simulink model "MutantsModel2"  (R2017b)
settings: Solver=ode3  StartTime=0.0  StopTime=inf  FixedStep=ts  RelTol=0.01  EnableMultiTasking=on
InitFcn:
  | ts=0.0005
  | %ts=100e-6;
StartFcn:
  | close all
StopFcn:
  | % Speed Torque Characterstic
  | 
  | 
  | %figure('Units','pixels', ...
  | %'Color',[1 1 1], ...
  | %'Name','Speed Torque Characterstic',...
  | %'NumberTitle','off',...
  | %'Position',[400 50 470 300], ...
  | %'ToolBar','none');
  | 
  | 
  | 
  | %plot(N_pi,Te_pi)
  | %title('Speed Torque Characterstic')
  | %xlabel('Speed [ RPM ]')
  | %ylabel('Electromagnetic Te_pi [ Nm ] ')
  | %grid on
  | %clear p4 p7 param5 param6 param8 parametres visible voltage
  | 
  | 
  | %clc
values from neighbouring files (symbols this model uses):
  TestOrder = [i]    [ExecuteTestSuite.m]    (also in mutants.m)
undefined symbols (not defined in the file or in its folder): emergency_button2, emergency_buttons, tc_simul, tc_size, temperature, trans1, trans2, trans3, trans4
libraries: simulink x44, powerlib_extras x11
(part 2 of 5)

== system MutantsModel2/mutant1/PI Control1 ==
  N* : Inport
  N : Inport  Port=2
  Abs : Abs  SaturateOnIntegerOverflow=on
  Abs1 : Abs  SaturateOnIntegerOverflow=on
  Abs2 : Abs
  Compare To Constant : simulink/Logic and Bit Operations/Compare To Constant  relop=<=  const=0.1  OutDataTypeStr=uint8
  Constant : Constant  Value=0
  Divide : Product  Inputs=/*
  Integrator Limited : Integrator  LimitOutput=on  UpperSaturationLimit=30  LowerSaturationLimit=-30
  Proportional gain : Gain  Gain=0.8  SaturateOnIntegerOverflow=on  OutDataTypeStr=Inherit: Same as input  ParamDataTypeStr=Inherit: Same as input
  Rate Transition3 : RateTransition  OutPortSampleTimeOpt=Inherit
  Saturation : Saturate  UpperLimit=inf  LowerLimit=2
  Saturation2 : Saturate  UpperLimit=120  LowerLimit=0.02
  Sum1 : Sum  Inputs=|+-  SaturateOnIntegerOverflow=on  InputSameDT=on  OutDataTypeStr=Inherit: Same as first input
  Sum2 : Sum  SaturateOnIntegerOverflow=on  InputSameDT=on  OutDataTypeStr=Inherit: Same as first input
  Sum3 : Sum  Inputs=|++  SaturateOnIntegerOverflow=on  InputSameDT=on  OutDataTypeStr=Inherit: Same as first input
  Switch : Switch  Threshold=0.5
  ctrl_sat : Saturate  UpperLimit=30  LowerLimit=-30
  rpm2hz : Gain  Gain=4/120  SaturateOnIntegerOverflow=on  OutDataTypeStr=Inherit: Same as input  ParamDataTypeStr=Inherit: Same as input
  "rpm2hz  " : Gain  Gain=4/120  SaturateOnIntegerOverflow=on  OutDataTypeStr=Inherit: Same as input  ParamDataTypeStr=Inherit: Same as input
  Freq* : Outport
  wires:
  N*/1 -> rpm2hz/1
  Sum2/1 -> ctrl_sat/1
  Sum3/1 -> Saturation2/1
  ctrl_sat/1 -> Sum3/1
  rpm2hz/1 -> Abs/1
  Proportional gain/1 -> Sum2/2
  "rpm2hz  "/1 -> Abs1/1
  Saturation2/1 -> Rate Transition3/1
  Sum1/1 -> Proportional gain/1, Switch/1, Abs2/1
  Abs/1 -> Saturation/1, Sum1/1
  Rate Transition3/1 -> Freq*/1
  Abs1/1 -> Sum3/2, Sum1/2
  N/1 -> "rpm2hz  "/1
  Integrator Limited/1 -> Sum2/1
  Divide/1 -> Compare To Constant/1
  Abs2/1 -> Divide/2
  Compare To Constant/1 -> Switch/2
  Constant/1 -> Switch/3
  Switch/1 -> Integrator Limited/1
  Saturation/1 -> Divide/1

== system MutantsModel2/mutant1/Subsystem ==
  Speed : Inport
  EmergButton1 : Inport  Port=2
  EmergButton2 : Inport  Port=3
  Temperature : Inport  Port=4
  Compare To Constant : simulink/Logic and Bit Operations/Compare To Constant  relop=>  const=100  OutDataTypeStr=boolean
  Compare To Constant1 : simulink/Logic and Bit Operations/Compare To Constant  relop===  const=0  OutDataTypeStr=boolean
  Constant : Constant  Value=emergency_buttons
  Constant1 : Constant  Value=temperature
  Constant2 : Constant  Value=emergency_button2
  Ir_a3 : Scope
  Logical Operator : Logic  Operator=OR  AllPortsSameDT=off  OutDataTypeStr=boolean
  Logical Operator1 : Logic  AllPortsSameDT=off  OutDataTypeStr=boolean
  Logical Operator2 : Logic  AllPortsSameDT=off  OutDataTypeStr=boolean
  Logical Operator3 : Logic  AllPortsSameDT=off  OutDataTypeStr=boolean
  Speed_to_0 : Constant  Value=0
  Switch : Switch  Criteria=u2 ~= 0
  Switch1 : Switch  Criteria=u2 ~= 0
  Switch2 : Switch  Criteria=u2 ~= 0
  Transfer Fcn1 : TransferFcn  Denominator=[10 1]
  "MotorSpeed " : Outport
  wires:
  Transfer Fcn1/1 -> Switch/3
  Compare To Constant1/1 -> Switch2/2
  Switch2/1 -> "MotorSpeed "/1, Ir_a3/1
  Switch1/1 -> Compare To Constant1/1, Switch2/1, Switch2/3
  Constant2/1 -> Logical Operator3/2
  Logical Operator3/1 -> Logical Operator/2
  Logical Operator2/1 -> Switch1/2
  Constant1/1 -> Logical Operator2/2
  Compare To Constant/1 -> Logical Operator2/1
  Temperature/1 -> Compare To Constant/1
  Constant/1 -> Logical Operator1/2
  Logical Operator1/1 -> Switch/2
  Speed_to_0/1 -> Switch/1, Switch1/1
  Switch/1 -> Switch1/3
  Speed/1 -> Transfer Fcn1/1
  Logical Operator/1 -> Logical Operator1/1
  EmergButton2/1 -> Logical Operator3/1
  EmergButton1/1 -> Logical Operator/1

== system MutantsModel2/mutant1/VSI ==
  Freq : Inport
  Fcn : Fcn  Expr=(2*sqrt(2/3)*Vdc/3)*(2*u(1)-u(2)-u(3))
  Fcn1 : Fcn  Expr=(2*sqrt(2/3)*Vdc/3)*(2*u(2)-u(3)-u(1))
  Fcn2 : Fcn  Expr=(2*sqrt(2/3)*Vdc/3)*(2*u(3)-u(2)-u(1))
  SPWM : Subsystem
  Va : Outport
  Vb : Outport  Port=2
  Vc : Outport  Port=3
  wires:
  Freq/1 -> SPWM/1(Freq)
  Fcn/1 -> Va/1
  Fcn2/1 -> Vc/1
  Fcn1/1 -> Vb/1
  SPWM/1(g) -> Fcn1/1, Fcn/1, Fcn2/1

== system MutantsModel2/mutant10/1 HP , 220 V Induction Motor ==
  tau : Inport
  V_a : Inport  Port=2
  V_b : Inport  Port=3
  V_c : Inport  Port=4
  Flux : Subsystem
  Measurements : Subsystem
  Mechanical : Subsystem
  Mux : Mux  Inputs=3
  Mux1 : Mux  Inputs=3
  abc to dq : Subsystem
  d_block : Subsystem
  dq to abc : Subsystem
  "dq to abc " : Subsystem
  q_block : Subsystem
  rad2rpm : Gain  Gain=30/pi
  m : Outport
  wires:
  Measurements/1(m) -> m/1
  rad2rpm/1 -> Measurements/8(N)
  Mux1/1 -> Measurements/2(I_r)
  Mux/1 -> Measurements/1(I_s)
  "dq to abc "/2(i_rb) -> Mux1/2
  "dq to abc "/3(i_rc) -> Mux1/3
  dq to abc/3(i_sc) -> Mux/3
  dq to abc/2(i_sb) -> Mux/2
  "dq to abc "/1(i_ra) -> Mux1/1
  dq to abc/1(i_sa) -> Mux/1
  V_a/1 -> abc to dq/1(Va)
  V_b/1 -> abc to dq/2(Vb)
  V_c/1 -> abc to dq/3(Vc)
  abc to dq/2(V_qs) -> Flux/2(V_qs)
  abc to dq/1(V_ds) -> Flux/1(V_ds)
  Flux/3(shi_qs) -> Mechanical/2(shi_qs), q_block/1(shi_qs)
  Flux/2("shi_dr ") -> d_block/2(shi_dr)
  tau/1 -> Mechanical/5(tau)
  Mechanical/1(Te) -> Measurements/7(Te)
  q_block/1(i_qs) -> Flux/5(I_qs), dq to abc/2(I_q), Measurements/5(I_qs), Measurements/4(I_dr), Mechanical/4(i_qs)
  q_block/2(i_qr) -> Flux/6(I_qr), "dq to abc "/2(I_q), Measurements/6(I_qr)
  d_block/2(i_dr) -> "dq to abc "/1(I_d), Flux/4(I_dr)
  d_block/1(i_ds) -> Flux/3(I_ds), dq to abc/1(I_d), Measurements/3(I_ds), Mechanical/3(i_ds)
  Flux/4("shi_qr ") -> q_block/2(shi_qr)
  Flux/1(shi_ds) -> Mechanical/1(shi_ds), d_block/1(shi_ds)
  Mechanical/3(we) -> Flux/7(we)
  Mechanical/2(omegaR) -> rad2rpm/1

== system MutantsModel2/mutant10/Data Acquision ==
  note: DONE TO HAVE AN ALLOWABLE SIMULATION TIME
  m : Inport
  speed : Inport  Port=2
  2nd-Order Filter : powerlib_extras/Control  Blocks/2nd-Order Filter  FilterType=Lowpass  Fo=120  Zeta=0.707  Initialize=off  Vac_Init=[1 45 60]  Vdc_Init=-0.5  PlotResponse=off  param1=[1 500 1]
  Bus Selector : BusSelector  OutputSignals=Mechanical.Rotor Speed in (rpm),Mechanical.Electromagnetic Torque (N*m),Stator Measurement.Stator Current i_sa (A)
  Mux : Mux  Inputs=2
  filtroPasaBajos : TransferFcn  Denominator=[1 1]
  is_a : Outport
  Te(Nm) : Outport  Port=2
  wm : Outport  Port=3
  wm1 : Outport  Port=4
  wires:
  filtroPasaBajos/1 -> Mux/1, wm1/1
  Mux/1 -> wm/1
  speed/1 -> Mux/2
  Bus Selector/3 -> is_a/1  "<Stator Current i_sa (A)>"
  Bus Selector/1 -> filtroPasaBajos/1  "<Rotor Speed in (rpm)>"
  m/1 -> Bus Selector/1
  Bus Selector/2 -> 2nd-Order Filter/1  "<Electromagnetic Torque (N*m)>"
  2nd-Order Filter/1 -> Te(Nm)/1

== system MutantsModel2/mutant10/PI Control1 ==
  N* : Inport
  N : Inport  Port=2
  Abs : Abs  SaturateOnIntegerOverflow=on
  Abs1 : Abs  SaturateOnIntegerOverflow=on
  Abs2 : Abs
  Compare To Constant : simulink/Logic and Bit Operations/Compare To Constant  relop=<=  const=0.1  OutDataTypeStr=uint8
  Constant : Constant  Value=0
  Divide : Product  Inputs=/*
  Integrator Limited : Integrator  LimitOutput=on  UpperSaturationLimit=30  LowerSaturationLimit=-30
  Proportional gain : Gain  Gain=0.8  SaturateOnIntegerOverflow=on  OutDataTypeStr=Inherit: Same as input  ParamDataTypeStr=Inherit: Same as input
  Rate Transition3 : RateTransition  OutPortSampleTimeOpt=Inherit
  Saturation : Saturate  UpperLimit=inf  LowerLimit=2
  Saturation2 : Saturate  UpperLimit=120  LowerLimit=0.02
  Sum1 : Sum  Inputs=|+-  SaturateOnIntegerOverflow=on  InputSameDT=on  OutDataTypeStr=Inherit: Same as first input
  Sum2 : Sum  SaturateOnIntegerOverflow=on  InputSameDT=on  OutDataTypeStr=Inherit: Same as first input
  Sum3 : Sum  Inputs=|++  SaturateOnIntegerOverflow=on  InputSameDT=on  OutDataTypeStr=Inherit: Same as first input
  Switch : Switch  Threshold=0.5
  ctrl_sat : Saturate  UpperLimit=30  LowerLimit=-30
  rpm2hz : Gain  Gain=4/120  SaturateOnIntegerOverflow=on  OutDataTypeStr=Inherit: Same as input  ParamDataTypeStr=Inherit: Same as input
  "rpm2hz  " : Gain  Gain=4/120  SaturateOnIntegerOverflow=on  OutDataTypeStr=Inherit: Same as input  ParamDataTypeStr=Inherit: Same as input
  Freq* : Outport
  wires:
  N*/1 -> rpm2hz/1
  Sum2/1 -> ctrl_sat/1
  Sum3/1 -> Saturation2/1
  ctrl_sat/1 -> Sum3/1
  rpm2hz/1 -> Abs/1
  Proportional gain/1 -> Sum2/2
  "rpm2hz  "/1 -> Abs1/1
  Saturation2/1 -> Rate Transition3/1
  Sum1/1 -> Proportional gain/1, Switch/1, Abs2/1
  Abs/1 -> Saturation/1, Sum1/1
  Rate Transition3/1 -> Freq*/1
  Abs1/1 -> Sum3/2, Sum1/2
  N/1 -> "rpm2hz  "/1
  Integrator Limited/1 -> Sum2/1
  Divide/1 -> Compare To Constant/1
  Abs2/1 -> Divide/2
  Compare To Constant/1 -> Switch/2
  Constant/1 -> Switch/3
  Switch/1 -> Integrator Limited/1
  Saturation/1 -> Divide/1

== system MutantsModel2/mutant10/Subsystem ==
  Speed : Inport
  EmergButton1 : Inport  Port=2
  EmergButton2 : Inport  Port=3
  Temperature : Inport  Port=4
  Compare To Constant : simulink/Logic and Bit Operations/Compare To Constant  relop=>  const=100  OutDataTypeStr=boolean
  Compare To Constant1 : simulink/Logic and Bit Operations/Compare To Constant  relop===  const=0  OutDataTypeStr=boolean
  Constant : Constant  Value=emergency_buttons
  Constant1 : Constant  Value=temperature
  Constant2 : Constant  Value=emergency_button2
  Ir_a3 : Scope
  Logical Operator : Logic  Operator=OR  AllPortsSameDT=off  OutDataTypeStr=boolean
  Logical Operator1 : Logic  Operator=NAND  AllPortsSameDT=off  OutDataTypeStr=boolean
  Logical Operator2 : Logic  AllPortsSameDT=off  OutDataTypeStr=boolean
  Logical Operator3 : Logic  AllPortsSameDT=off  OutDataTypeStr=boolean
  Speed_to_0 : Constant  Value=0
  Switch : Switch  Criteria=u2 ~= 0
  Switch1 : Switch  Criteria=u2 ~= 0
  Switch2 : Switch  Criteria=u2 ~= 0
  Transfer Fcn1 : TransferFcn  Denominator=[20 1]
  "MotorSpeed " : Outport
  wires:
  Transfer Fcn1/1 -> Switch/3
  Compare To Constant1/1 -> Switch2/2
  Switch2/1 -> "MotorSpeed "/1, Ir_a3/1
  Switch1/1 -> Compare To Constant1/1, Switch2/1, Switch2/3
  Constant2/1 -> Logical Operator3/2
  Logical Operator3/1 -> Logical Operator/2
  Logical Operator2/1 -> Switch1/2
  Constant1/1 -> Logical Operator2/2
  Compare To Constant/1 -> Logical Operator2/1
  Temperature/1 -> Compare To Constant/1
  Constant/1 -> Logical Operator1/2
  Logical Operator1/1 -> Switch/2
  Speed_to_0/1 -> Switch/1, Switch1/1
  Switch/1 -> Switch1/3
  Speed/1 -> Transfer Fcn1/1
  Logical Operator/1 -> Logical Operator1/1
  EmergButton2/1 -> Logical Operator3/1
  EmergButton1/1 -> Logical Operator/1

== system MutantsModel2/mutant10/VSI ==
  Freq : Inport
  Fcn : Fcn  Expr=(2*sqrt(2/3)*Vdc/3)*(2*u(1)-u(2)-u(3))
  Fcn1 : Fcn  Expr=(2*sqrt(2/3)*Vdc/3)*(2*u(2)-u(3)-u(1))
  Fcn2 : Fcn  Expr=(2*sqrt(2/3)*Vdc/3)*(2*u(3)-u(2)-u(1))
  SPWM : Subsystem
  Va : Outport
  Vb : Outport  Port=2
  Vc : Outport  Port=3
  wires:
  Freq/1 -> SPWM/1(Freq)
  Fcn/1 -> Va/1
  Fcn2/1 -> Vc/1
  Fcn1/1 -> Vb/1
  SPWM/1(g) -> Fcn1/1, Fcn/1, Fcn2/1

== system MutantsModel2/mutant2/1 HP , 220 V Induction Motor ==
  tau : Inport
  V_a : Inport  Port=2
  V_b : Inport  Port=3
  V_c : Inport  Port=4
  Flux : Subsystem
  Measurements : Subsystem
  Mechanical : Subsystem
  Mux : Mux  Inputs=3
  Mux1 : Mux  Inputs=3
  abc to dq : Subsystem
  d_block : Subsystem
  dq to abc : Subsystem
  "dq to abc " : Subsystem
  q_block : Subsystem
  rad2rpm : Gain  Gain=30/pi
  m : Outport
  wires:
  Mechanical/2(omegaR) -> rad2rpm/1
  Mechanical/3(we) -> Flux/7(we)
  Flux/1(shi_ds) -> d_block/1(shi_ds), Mechanical/1(shi_ds)
  Flux/4("shi_qr ") -> q_block/2(shi_qr)
  d_block/1(i_ds) -> Mechanical/3(i_ds), Measurements/3(I_ds), dq to abc/1(I_d), Flux/3(I_ds)
  d_block/2(i_dr) -> Flux/4(I_dr), "dq to abc "/1(I_d)
  q_block/2(i_qr) -> Measurements/6(I_qr), "dq to abc "/2(I_q), Flux/6(I_qr)
  q_block/1(i_qs) -> Mechanical/4(i_qs), Measurements/4(I_dr), Measurements/5(I_qs), dq to abc/2(I_q), Flux/5(I_qs)
  Mechanical/1(Te) -> Measurements/7(Te)
  tau/1 -> Mechanical/5(tau)
  Flux/2("shi_dr ") -> d_block/2(shi_dr)
  Flux/3(shi_qs) -> q_block/1(shi_qs), Mechanical/2(shi_qs)
  abc to dq/1(V_ds) -> Flux/1(V_ds)
  abc to dq/2(V_qs) -> Flux/2(V_qs)
  V_c/1 -> abc to dq/3(Vc)
  V_b/1 -> abc to dq/2(Vb)
  V_a/1 -> abc to dq/1(Va)
  dq to abc/1(i_sa) -> Mux/1
  "dq to abc "/1(i_ra) -> Mux1/1
  dq to abc/2(i_sb) -> Mux/2
  dq to abc/3(i_sc) -> Mux/3
  "dq to abc "/3(i_rc) -> Mux1/3
  "dq to abc "/2(i_rb) -> Mux1/2
  Mux/1 -> Measurements/1(I_s)
  Mux1/1 -> Measurements/2(I_r)
  rad2rpm/1 -> Measurements/8(N)
  Measurements/1(m) -> m/1

== system MutantsModel2/mutant2/Data Acquision ==
  note: DONE TO HAVE AN ALLOWABLE SIMULATION TIME
  m : Inport
  speed : Inport  Port=2
  2nd-Order Filter : powerlib_extras/Control  Blocks/2nd-Order Filter  FilterType=Lowpass  Fo=120  Zeta=0.707  Initialize=off  Vac_Init=[1 45 60]  Vdc_Init=-0.5  PlotResponse=off  param1=[1 500 1]
  Bus Selector : BusSelector  OutputSignals=Mechanical.Rotor Speed in (rpm),Mechanical.Electromagnetic Torque (N*m),Stator Measurement.Stator Current i_sa (A)
  Mux : Mux  Inputs=2
  filtroPasaBajos : TransferFcn  Denominator=[1 1]
  is_a : Outport
  Te(Nm) : Outport  Port=2
  wm : Outport  Port=3
  wm1 : Outport  Port=4
  wires:
  2nd-Order Filter/1 -> Te(Nm)/1
  Bus Selector/2 -> 2nd-Order Filter/1  "<Electromagnetic Torque (N*m)>"
  m/1 -> Bus Selector/1
  Bus Selector/1 -> filtroPasaBajos/1  "<Rotor Speed in (rpm)>"
  Bus Selector/3 -> is_a/1  "<Stator Current i_sa (A)>"
  speed/1 -> Mux/2
  Mux/1 -> wm/1
  filtroPasaBajos/1 -> wm1/1, Mux/1

== system MutantsModel2/mutant2/PI Control1 ==
  N* : Inport
  N : Inport  Port=2
  Abs : Abs  SaturateOnIntegerOverflow=on
  Abs1 : Abs  SaturateOnIntegerOverflow=on
  Abs2 : Abs
  Compare To Constant : simulink/Logic and Bit Operations/Compare To Constant  relop=<=  const=0.1  OutDataTypeStr=uint8
  Constant : Constant  Value=0
  Divide : Product  Inputs=/*
  Integrator Limited : Integrator  LimitOutput=on  UpperSaturationLimit=30  LowerSaturationLimit=-30
  Proportional gain : Gain  Gain=0.8  SaturateOnIntegerOverflow=on  OutDataTypeStr=Inherit: Same as input  ParamDataTypeStr=Inherit: Same as input
  Rate Transition3 : RateTransition  OutPortSampleTimeOpt=Inherit
  Saturation : Saturate  UpperLimit=inf  LowerLimit=2
  Saturation2 : Saturate  UpperLimit=120  LowerLimit=0.02
  Sum1 : Sum  Inputs=|+-  SaturateOnIntegerOverflow=on  InputSameDT=on  OutDataTypeStr=Inherit: Same as first input
  Sum2 : Sum  SaturateOnIntegerOverflow=on  InputSameDT=on  OutDataTypeStr=Inherit: Same as first input
  Sum3 : Sum  Inputs=|++  SaturateOnIntegerOverflow=on  InputSameDT=on  OutDataTypeStr=Inherit: Same as first input
  Switch : Switch  Threshold=0.5
  ctrl_sat : Saturate  UpperLimit=30  LowerLimit=-30
  rpm2hz : Gain  Gain=4/120  SaturateOnIntegerOverflow=on  OutDataTypeStr=Inherit: Same as input  ParamDataTypeStr=Inherit: Same as input
  "rpm2hz  " : Gain  Gain=4/120  SaturateOnIntegerOverflow=on  OutDataTypeStr=Inherit: Same as input  ParamDataTypeStr=Inherit: Same as input
  Freq* : Outport
  wires:
  Saturation/1 -> Divide/1
  Switch/1 -> Integrator Limited/1
  Constant/1 -> Switch/3
  Compare To Constant/1 -> Switch/2
  Abs2/1 -> Divide/2
  Divide/1 -> Compare To Constant/1
  Integrator Limited/1 -> Sum2/1
  N/1 -> "rpm2hz  "/1
  Abs1/1 -> Sum1/2, Sum3/2
  Rate Transition3/1 -> Freq*/1
  Abs/1 -> Sum1/1, Saturation/1
  Sum1/1 -> Abs2/1, Switch/1, Proportional gain/1
  Saturation2/1 -> Rate Transition3/1
  "rpm2hz  "/1 -> Abs1/1
  Proportional gain/1 -> Sum2/2
  rpm2hz/1 -> Abs/1
  ctrl_sat/1 -> Sum3/1
  Sum3/1 -> Saturation2/1
  Sum2/1 -> ctrl_sat/1
  N*/1 -> rpm2hz/1

== system MutantsModel2/mutant2/Subsystem ==
  Speed : Inport
  EmergButton1 : Inport  Port=2
  EmergButton2 : Inport  Port=3
  Temperature : Inport  Port=4
  Compare To Constant : simulink/Logic and Bit Operations/Compare To Constant  relop=>  const=70  OutDataTypeStr=boolean
  Compare To Constant1 : simulink/Logic and Bit Operations/Compare To Constant  relop===  const=0  OutDataTypeStr=boolean
  Constant : Constant  Value=emergency_buttons
  Constant1 : Constant  Value=temperature
  Constant2 : Constant  Value=emergency_button2
  Ir_a3 : Scope
  Logical Operator : Logic  Operator=OR  AllPortsSameDT=off  OutDataTypeStr=boolean
  Logical Operator1 : Logic  AllPortsSameDT=off  OutDataTypeStr=boolean
  Logical Operator2 : Logic  AllPortsSameDT=off  OutDataTypeStr=boolean
  Logical Operator3 : Logic  AllPortsSameDT=off  OutDataTypeStr=boolean
  Speed_to_0 : Constant  Value=0
  Switch : Switch  Criteria=u2 ~= 0
  Switch1 : Switch  Criteria=u2 ~= 0
  Switch2 : Switch  Criteria=u2 ~= 0
  Transfer Fcn1 : TransferFcn  Denominator=[20 1]
  "MotorSpeed " : Outport
  wires:
  EmergButton1/1 -> Logical Operator/1
  EmergButton2/1 -> Logical Operator3/1
  Logical Operator/1 -> Logical Operator1/1
  Speed/1 -> Transfer Fcn1/1
  Switch/1 -> Switch1/3
  Speed_to_0/1 -> Switch1/1, Switch/1
  Logical Operator1/1 -> Switch/2
  Constant/1 -> Logical Operator1/2
  Temperature/1 -> Compare To Constant/1
  Compare To Constant/1 -> Logical Operator2/1
  Constant1/1 -> Logical Operator2/2
  Logical Operator2/1 -> Switch1/2
  Logical Operator3/1 -> Logical Operator/2
  Constant2/1 -> Logical Operator3/2
  Switch1/1 -> Switch2/3, Switch2/1, Compare To Constant1/1
  Switch2/1 -> Ir_a3/1, "MotorSpeed "/1
  Compare To Constant1/1 -> Switch2/2
  Transfer Fcn1/1 -> Switch/3

== system MutantsModel2/mutant2/VSI ==
  Freq : Inport
  Fcn : Fcn  Expr=(2*sqrt(2/3)*Vdc/3)*(2*u(1)-u(2)-u(3))
  Fcn1 : Fcn  Expr=(2*sqrt(2/3)*Vdc/3)*(2*u(2)-u(3)-u(1))
  Fcn2 : Fcn  Expr=(2*sqrt(2/3)*Vdc/3)*(2*u(3)-u(2)-u(1))
  SPWM : Subsystem
  Va : Outport
  Vb : Outport  Port=2
  Vc : Outport  Port=3
  wires:
  SPWM/1(g) -> Fcn2/1, Fcn/1, Fcn1/1
  Fcn1/1 -> Vb/1
  Fcn2/1 -> Vc/1
  Fcn/1 -> Va/1
  Freq/1 -> SPWM/1(Freq)

== system MutantsModel2/mutant3/1 HP , 220 V Induction Motor ==
  tau : Inport
  V_a : Inport  Port=2
  V_b : Inport  Port=3
  V_c : Inport  Port=4
  Flux : Subsystem
  Measurements : Subsystem
  Mechanical : Subsystem
  Mux : Mux  Inputs=3
  Mux1 : Mux  Inputs=3
  abc to dq : Subsystem
  d_block : Subsystem
  dq to abc : Subsystem
  "dq to abc " : Subsystem
  q_block : Subsystem
  rad2rpm : Gain  Gain=30/pi
  m : Outport
  wires:
  Measurements/1(m) -> m/1
  rad2rpm/1 -> Measurements/8(N)
  Mux1/1 -> Measurements/2(I_r)
  Mux/1 -> Measurements/1(I_s)
  "dq to abc "/2(i_rb) -> Mux1/2
  "dq to abc "/3(i_rc) -> Mux1/3
  dq to abc/3(i_sc) -> Mux/3
  dq to abc/2(i_sb) -> Mux/2
  "dq to abc "/1(i_ra) -> Mux1/1
  dq to abc/1(i_sa) -> Mux/1
  V_a/1 -> abc to dq/1(Va)
  V_b/1 -> abc to dq/2(Vb)
  V_c/1 -> abc to dq/3(Vc)
  abc to dq/2(V_qs) -> Flux/2(V_qs)
  abc to dq/1(V_ds) -> Flux/1(V_ds)
  Flux/3(shi_qs) -> Mechanical/2(shi_qs), q_block/1(shi_qs)
  Flux/2("shi_dr ") -> d_block/2(shi_dr)
  tau/1 -> Mechanical/5(tau)
  Mechanical/1(Te) -> Measurements/7(Te)
  q_block/1(i_qs) -> Flux/5(I_qs), dq to abc/2(I_q), Measurements/5(I_qs), Measurements/4(I_dr), Mechanical/4(i_qs)
  q_block/2(i_qr) -> Flux/6(I_qr), "dq to abc "/2(I_q), Measurements/6(I_qr)
  d_block/2(i_dr) -> "dq to abc "/1(I_d), Flux/4(I_dr)
  d_block/1(i_ds) -> Flux/3(I_ds), dq to abc/1(I_d), Measurements/3(I_ds), Mechanical/3(i_ds)
  Flux/4("shi_qr ") -> q_block/2(shi_qr)
  Flux/1(shi_ds) -> Mechanical/1(shi_ds), d_block/1(shi_ds)
  Mechanical/3(we) -> Flux/7(we)
  Mechanical/2(omegaR) -> rad2rpm/1

== system MutantsModel2/mutant3/Data Acquision ==
  note: DONE TO HAVE AN ALLOWABLE SIMULATION TIME
  m : Inport
  speed : Inport  Port=2
  2nd-Order Filter : powerlib_extras/Control  Blocks/2nd-Order Filter  FilterType=Lowpass  Fo=120  Zeta=0.707  Initialize=off  Vac_Init=[1 45 60]  Vdc_Init=-0.5  PlotResponse=off  param1=[1 500 1]
  Bus Selector : BusSelector  OutputSignals=Mechanical.Rotor Speed in (rpm),Mechanical.Electromagnetic Torque (N*m),Stator Measurement.Stator Current i_sa (A)
  Mux : Mux  Inputs=2
  filtroPasaBajos : TransferFcn  Denominator=[1 1]
  is_a : Outport
  Te(Nm) : Outport  Port=2
  wm : Outport  Port=3
  wm1 : Outport  Port=4
  wires:
  filtroPasaBajos/1 -> Mux/1, wm1/1
  Mux/1 -> wm/1
  speed/1 -> Mux/2
  Bus Selector/3 -> is_a/1  "<Stator Current i_sa (A)>"
  Bus Selector/1 -> filtroPasaBajos/1  "<Rotor Speed in (rpm)>"
  m/1 -> Bus Selector/1
  Bus Selector/2 -> 2nd-Order Filter/1  "<Electromagnetic Torque (N*m)>"
  2nd-Order Filter/1 -> Te(Nm)/1

== system MutantsModel2/mutant3/PI Control1 ==
  N* : Inport
  N : Inport  Port=2
  Abs : Abs  SaturateOnIntegerOverflow=on
  Abs1 : Abs  SaturateOnIntegerOverflow=on
  Abs2 : Abs
  Compare To Constant : simulink/Logic and Bit Operations/Compare To Constant  relop=<=  const=0.1  OutDataTypeStr=uint8
  Constant : Constant  Value=0
  Divide : Product  Inputs=/*
  Integrator Limited : Integrator  LimitOutput=on  UpperSaturationLimit=30  LowerSaturationLimit=-30
  Proportional gain : Gain  Gain=0.8  SaturateOnIntegerOverflow=on  OutDataTypeStr=Inherit: Same as input  ParamDataTypeStr=Inherit: Same as input
  Rate Transition3 : RateTransition  OutPortSampleTimeOpt=Inherit
  Saturation : Saturate  UpperLimit=inf  LowerLimit=2
  Saturation2 : Saturate  UpperLimit=120  LowerLimit=0.02
  Sum1 : Sum  Inputs=|+-  SaturateOnIntegerOverflow=on  InputSameDT=on  OutDataTypeStr=Inherit: Same as first input
  Sum2 : Sum  SaturateOnIntegerOverflow=on  InputSameDT=on  OutDataTypeStr=Inherit: Same as first input
  Sum3 : Sum  Inputs=|++  SaturateOnIntegerOverflow=on  InputSameDT=on  OutDataTypeStr=Inherit: Same as first input
  Switch : Switch  Threshold=0.5
  ctrl_sat : Saturate  UpperLimit=30  LowerLimit=-30
  rpm2hz : Gain  Gain=4/120  SaturateOnIntegerOverflow=on  OutDataTypeStr=Inherit: Same as input  ParamDataTypeStr=Inherit: Same as input
  "rpm2hz  " : Gain  Gain=4/120  SaturateOnIntegerOverflow=on  OutDataTypeStr=Inherit: Same as input  ParamDataTypeStr=Inherit: Same as input
  Freq* : Outport
  wires:
  N*/1 -> rpm2hz/1
  Sum2/1 -> ctrl_sat/1
  Sum3/1 -> Saturation2/1
  ctrl_sat/1 -> Sum3/1
  rpm2hz/1 -> Abs/1
  Proportional gain/1 -> Sum2/2
  "rpm2hz  "/1 -> Abs1/1
  Saturation2/1 -> Rate Transition3/1
  Sum1/1 -> Proportional gain/1, Switch/1, Abs2/1
  Abs/1 -> Saturation/1, Sum1/1
  Rate Transition3/1 -> Freq*/1
  Abs1/1 -> Sum3/2, Sum1/2
  N/1 -> "rpm2hz  "/1
  Integrator Limited/1 -> Sum2/1
  Divide/1 -> Compare To Constant/1
  Abs2/1 -> Divide/2
  Compare To Constant/1 -> Switch/2
  Constant/1 -> Switch/3
  Switch/1 -> Integrator Limited/1
  Saturation/1 -> Divide/1

== system MutantsModel2/mutant3/Subsystem ==
  Speed : Inport
  EmergButton1 : Inport  Port=2
  EmergButton2 : Inport  Port=3
  Temperature : Inport  Port=4
  Compare To Constant : simulink/Logic and Bit Operations/Compare To Constant  relop=>  const=100  OutDataTypeStr=boolean
  Compare To Constant1 : simulink/Logic and Bit Operations/Compare To Constant  relop===  const=0  OutDataTypeStr=boolean
  Constant : Constant  Value=emergency_buttons
  Constant1 : Constant  Value=temperature
  Constant2 : Constant  Value=emergency_button2
  Ir_a3 : Scope
  Logical Operator{,1..3} (4 alike) : Logic  AllPortsSameDT=off  OutDataTypeStr=boolean
  Speed_to_0 : Constant  Value=0
  Switch : Switch  Criteria=u2 ~= 0
  Switch1 : Switch  Criteria=u2 ~= 0
  Switch2 : Switch  Criteria=u2 ~= 0
  Transfer Fcn1 : TransferFcn  Denominator=[20 1]
  "MotorSpeed " : Outport
  wires:
  Transfer Fcn1/1 -> Switch/3
  Compare To Constant1/1 -> Switch2/2
  Switch2/1 -> "MotorSpeed "/1, Ir_a3/1
  Switch1/1 -> Compare To Constant1/1, Switch2/1, Switch2/3
  Constant2/1 -> Logical Operator3/2
  Logical Operator3/1 -> Logical Operator/2
  Logical Operator2/1 -> Switch1/2
  Constant1/1 -> Logical Operator2/2
  Compare To Constant/1 -> Logical Operator2/1
  Temperature/1 -> Compare To Constant/1
  Constant/1 -> Logical Operator1/2
  Logical Operator1/1 -> Switch/2
  Speed_to_0/1 -> Switch/1, Switch1/1
  Switch/1 -> Switch1/3
  Speed/1 -> Transfer Fcn1/1
  Logical Operator/1 -> Logical Operator1/1
  EmergButton2/1 -> Logical Operator3/1
  EmergButton1/1 -> Logical Operator/1

== system MutantsModel2/mutant3/VSI ==
  Freq : Inport
  Fcn : Fcn  Expr=(2*sqrt(2/3)*Vdc/3)*(2*u(1)-u(2)-u(3))
  Fcn1 : Fcn  Expr=(2*sqrt(2/3)*Vdc/3)*(2*u(2)-u(3)-u(1))
  Fcn2 : Fcn  Expr=(2*sqrt(2/3)*Vdc/3)*(2*u(3)-u(2)-u(1))
  SPWM : Subsystem
  Va : Outport
  Vb : Outport  Port=2
  Vc : Outport  Port=3
  wires:
  Freq/1 -> SPWM/1(Freq)
  Fcn/1 -> Va/1
  Fcn2/1 -> Vc/1
  Fcn1/1 -> Vb/1
  SPWM/1(g) -> Fcn1/1, Fcn/1, Fcn2/1

== system MutantsModel2/mutant4/1 HP , 220 V Induction Motor ==
  tau : Inport
  V_a : Inport  Port=2
  V_b : Inport  Port=3
  V_c : Inport  Port=4
  Flux : Subsystem
  Measurements : Subsystem
  Mechanical : Subsystem
  Mux : Mux  Inputs=3
  Mux1 : Mux  Inputs=3
  abc to dq : Subsystem
  d_block : Subsystem
  dq to abc : Subsystem
  "dq to abc " : Subsystem
  q_block : Subsystem
  rad2rpm : Gain  Gain=30/pi
  m : Outport
  wires:
  Mechanical/2(omegaR) -> rad2rpm/1
  Mechanical/3(we) -> Flux/7(we)
  Flux/1(shi_ds) -> d_block/1(shi_ds), Mechanical/1(shi_ds)
  Flux/4("shi_qr ") -> q_block/2(shi_qr)
  d_block/1(i_ds) -> Mechanical/3(i_ds), Measurements/3(I_ds), dq to abc/1(I_d), Flux/3(I_ds)
  d_block/2(i_dr) -> Flux/4(I_dr), "dq to abc "/1(I_d)
  q_block/2(i_qr) -> Measurements/6(I_qr), "dq to abc "/2(I_q), Flux/6(I_qr)
  q_block/1(i_qs) -> Mechanical/4(i_qs), Measurements/4(I_dr), Measurements/5(I_qs), dq to abc/2(I_q), Flux/5(I_qs)
  Mechanical/1(Te) -> Measurements/7(Te)
  tau/1 -> Mechanical/5(tau)
  Flux/2("shi_dr ") -> d_block/2(shi_dr)
  Flux/3(shi_qs) -> q_block/1(shi_qs), Mechanical/2(shi_qs)
  abc to dq/1(V_ds) -> Flux/1(V_ds)
  abc to dq/2(V_qs) -> Flux/2(V_qs)
  V_c/1 -> abc to dq/3(Vc)
  V_b/1 -> abc to dq/2(Vb)
  V_a/1 -> abc to dq/1(Va)
  dq to abc/1(i_sa) -> Mux/1
  "dq to abc "/1(i_ra) -> Mux1/1
  dq to abc/2(i_sb) -> Mux/2
  dq to abc/3(i_sc) -> Mux/3
  "dq to abc "/3(i_rc) -> Mux1/3
  "dq to abc "/2(i_rb) -> Mux1/2
  Mux/1 -> Measurements/1(I_s)
  Mux1/1 -> Measurements/2(I_r)
  rad2rpm/1 -> Measurements/8(N)
  Measurements/1(m) -> m/1

== system MutantsModel2/mutant4/Data Acquision ==
  note: DONE TO HAVE AN ALLOWABLE SIMULATION TIME
  m : Inport
  speed : Inport  Port=2
  2nd-Order Filter : powerlib_extras/Control  Blocks/2nd-Order Filter  FilterType=Lowpass  Fo=120  Zeta=0.707  Initialize=off  Vac_Init=[1 45 60]  Vdc_Init=-0.5  PlotResponse=off  param1=[1 500 1]
  Bus Selector : BusSelector  OutputSignals=Mechanical.Rotor Speed in (rpm),Mechanical.Electromagnetic Torque (N*m),Stator Measurement.Stator Current i_sa (A)
  Mux : Mux  Inputs=2
  filtroPasaBajos : TransferFcn  Denominator=[1 1]
  is_a : Outport
  Te(Nm) : Outport  Port=2
  wm : Outport  Port=3
  wm1 : Outport  Port=4
  wires:
  2nd-Order Filter/1 -> Te(Nm)/1
  Bus Selector/2 -> 2nd-Order Filter/1  "<Electromagnetic Torque (N*m)>"
  m/1 -> Bus Selector/1
  Bus Selector/1 -> filtroPasaBajos/1  "<Rotor Speed in (rpm)>"
  Bus Selector/3 -> is_a/1  "<Stator Current i_sa (A)>"
  speed/1 -> Mux/2
  Mux/1 -> wm/1
  filtroPasaBajos/1 -> wm1/1, Mux/1

== system MutantsModel2/mutant4/PI Control1 ==
  N* : Inport
  N : Inport  Port=2
  Abs : Abs  SaturateOnIntegerOverflow=on
  Abs1 : Abs  SaturateOnIntegerOverflow=on
  Abs2 : Abs
  Compare To Constant : simulink/Logic and Bit Operations/Compare To Constant  relop=<=  const=0.1  OutDataTypeStr=uint8
  Constant : Constant  Value=0
  Divide : Product  Inputs=/*
  Integrator Limited : Integrator  LimitOutput=on  UpperSaturationLimit=30  LowerSaturationLimit=-30
  Proportional gain : Gain  Gain=0.8  SaturateOnIntegerOverflow=on  OutDataTypeStr=Inherit: Same as input  ParamDataTypeStr=Inherit: Same as input
  Rate Transition3 : RateTransition  OutPortSampleTimeOpt=Inherit
  Saturation : Saturate  UpperLimit=inf  LowerLimit=2
  Saturation2 : Saturate  UpperLimit=120  LowerLimit=0.02
  Sum1 : Sum  Inputs=|+-  SaturateOnIntegerOverflow=on  InputSameDT=on  OutDataTypeStr=Inherit: Same as first input
  Sum2 : Sum  SaturateOnIntegerOverflow=on  InputSameDT=on  OutDataTypeStr=Inherit: Same as first input
  Sum3 : Sum  Inputs=|++  SaturateOnIntegerOverflow=on  InputSameDT=on  OutDataTypeStr=Inherit: Same as first input
  Switch : Switch  Threshold=0.5
  ctrl_sat : Saturate  UpperLimit=30  LowerLimit=-30
  rpm2hz : Gain  Gain=4/120  SaturateOnIntegerOverflow=on  OutDataTypeStr=Inherit: Same as input  ParamDataTypeStr=Inherit: Same as input
  "rpm2hz  " : Gain  Gain=4/120  SaturateOnIntegerOverflow=on  OutDataTypeStr=Inherit: Same as input  ParamDataTypeStr=Inherit: Same as input
  Freq* : Outport
  wires:
  Saturation/1 -> Divide/1
  Switch/1 -> Integrator Limited/1
  Constant/1 -> Switch/3
  Compare To Constant/1 -> Switch/2
  Abs2/1 -> Divide/2
  Divide/1 -> Compare To Constant/1
  Integrator Limited/1 -> Sum2/1
  N/1 -> "rpm2hz  "/1
  Abs1/1 -> Sum1/2, Sum3/2
  Rate Transition3/1 -> Freq*/1
  Abs/1 -> Sum1/1, Saturation/1
  Sum1/1 -> Abs2/1, Switch/1, Proportional gain/1
  Saturation2/1 -> Rate Transition3/1
  "rpm2hz  "/1 -> Abs1/1
  Proportional gain/1 -> Sum2/2
  rpm2hz/1 -> Abs/1
  ctrl_sat/1 -> Sum3/1
  Sum3/1 -> Saturation2/1
  Sum2/1 -> ctrl_sat/1
  N*/1 -> rpm2hz/1

== system MutantsModel2/mutant4/Subsystem ==
  Speed : Inport
  EmergButton1 : Inport  Port=2
  EmergButton2 : Inport  Port=3
  Temperature : Inport  Port=4
  Compare To Constant : simulink/Logic and Bit Operations/Compare To Constant  relop=>  const=100  OutDataTypeStr=boolean
  Compare To Constant1 : simulink/Logic and Bit Operations/Compare To Constant  relop===  const=0  OutDataTypeStr=boolean
  Constant : Constant  Value=emergency_buttons
  Constant1 : Constant  Value=temperature
  Constant2 : Constant  Value=emergency_button2
  Ir_a3 : Scope
  Logical Operator : Logic  Operator=OR  AllPortsSameDT=off  OutDataTypeStr=boolean
  Logical Operator1 : Logic  AllPortsSameDT=off  OutDataTypeStr=boolean
  Logical Operator2 : Logic  Operator=OR  AllPortsSameDT=off  OutDataTypeStr=boolean
  Logical Operator3 : Logic  AllPortsSameDT=off  OutDataTypeStr=boolean
  Speed_to_0 : Constant  Value=0
  Switch : Switch  Criteria=u2 ~= 0
  Switch1 : Switch  Criteria=u2 ~= 0
  Switch2 : Switch  Criteria=u2 ~= 0
  Transfer Fcn1 : TransferFcn  Denominator=[20 1]
  "MotorSpeed " : Outport
  wires:
  EmergButton1/1 -> Logical Operator/1
  EmergButton2/1 -> Logical Operator3/1
  Logical Operator/1 -> Logical Operator1/1
  Speed/1 -> Transfer Fcn1/1
  Switch/1 -> Switch1/3
  Speed_to_0/1 -> Switch1/1, Switch/1
  Logical Operator1/1 -> Switch/2
  Constant/1 -> Logical Operator1/2
  Temperature/1 -> Compare To Constant/1
  Compare To Constant/1 -> Logical Operator2/1
  Constant1/1 -> Logical Operator2/2
  Logical Operator2/1 -> Switch1/2
  Logical Operator3/1 -> Logical Operator/2
  Constant2/1 -> Logical Operator3/2
  Switch1/1 -> Switch2/3, Switch2/1, Compare To Constant1/1
  Switch2/1 -> Ir_a3/1, "MotorSpeed "/1
  Compare To Constant1/1 -> Switch2/2
  Transfer Fcn1/1 -> Switch/3

== system MutantsModel2/mutant4/VSI ==
  Freq : Inport
  Fcn : Fcn  Expr=(2*sqrt(2/3)*Vdc/3)*(2*u(1)-u(2)-u(3))
  Fcn1 : Fcn  Expr=(2*sqrt(2/3)*Vdc/3)*(2*u(2)-u(3)-u(1))
  Fcn2 : Fcn  Expr=(2*sqrt(2/3)*Vdc/3)*(2*u(3)-u(2)-u(1))
  SPWM : Subsystem
  Va : Outport
  Vb : Outport  Port=2
  Vc : Outport  Port=3
  wires:
  SPWM/1(g) -> Fcn2/1, Fcn/1, Fcn1/1
  Fcn1/1 -> Vb/1
  Fcn2/1 -> Vc/1
  Fcn/1 -> Va/1
  Freq/1 -> SPWM/1(Freq)

== system MutantsModel2/mutant5/1 HP , 220 V Induction Motor ==
  tau : Inport
  V_a : Inport  Port=2
  V_b : Inport  Port=3
  V_c : Inport  Port=4
  Flux : Subsystem
  Measurements : Subsystem
  Mechanical : Subsystem
  Mux : Mux  Inputs=3
  Mux1 : Mux  Inputs=3
  abc to dq : Subsystem
  d_block : Subsystem
  dq to abc : Subsystem
  "dq to abc " : Subsystem
  q_block : Subsystem
  rad2rpm : Gain  Gain=30/pi
  m : Outport
  wires:
  Measurements/1(m) -> m/1
  rad2rpm/1 -> Measurements/8(N)
  Mux1/1 -> Measurements/2(I_r)
  Mux/1 -> Measurements/1(I_s)
  "dq to abc "/2(i_rb) -> Mux1/2
  "dq to abc "/3(i_rc) -> Mux1/3
  dq to abc/3(i_sc) -> Mux/3
  dq to abc/2(i_sb) -> Mux/2
  "dq to abc "/1(i_ra) -> Mux1/1
  dq to abc/1(i_sa) -> Mux/1
  V_a/1 -> abc to dq/1(Va)
  V_b/1 -> abc to dq/2(Vb)
  V_c/1 -> abc to dq/3(Vc)
  abc to dq/2(V_qs) -> Flux/2(V_qs)
  abc to dq/1(V_ds) -> Flux/1(V_ds)
  Flux/3(shi_qs) -> Mechanical/2(shi_qs), q_block/1(shi_qs)
  Flux/2("shi_dr ") -> d_block/2(shi_dr)
  tau/1 -> Mechanical/5(tau)
  Mechanical/1(Te) -> Measurements/7(Te)
  q_block/1(i_qs) -> Flux/5(I_qs), dq to abc/2(I_q), Measurements/5(I_qs), Measurements/4(I_dr), Mechanical/4(i_qs)
  q_block/2(i_qr) -> Flux/6(I_qr), "dq to abc "/2(I_q), Measurements/6(I_qr)
  d_block/2(i_dr) -> "dq to abc "/1(I_d), Flux/4(I_dr)
  d_block/1(i_ds) -> Flux/3(I_ds), dq to abc/1(I_d), Measurements/3(I_ds), Mechanical/3(i_ds)
  Flux/4("shi_qr ") -> q_block/2(shi_qr)
  Flux/1(shi_ds) -> Mechanical/1(shi_ds), d_block/1(shi_ds)
  Mechanical/3(we) -> Flux/7(we)
  Mechanical/2(omegaR) -> rad2rpm/1

== system MutantsModel2/mutant5/Data Acquision ==
  note: DONE TO HAVE AN ALLOWABLE SIMULATION TIME
  m : Inport
  speed : Inport  Port=2
  2nd-Order Filter : powerlib_extras/Control  Blocks/2nd-Order Filter  FilterType=Lowpass  Fo=120  Zeta=0.707  Initialize=off  Vac_Init=[1 45 60]  Vdc_Init=-0.5  PlotResponse=off  param1=[1 500 1]
  Bus Selector : BusSelector  OutputSignals=Mechanical.Rotor Speed in (rpm),Mechanical.Electromagnetic Torque (N*m),Stator Measurement.Stator Current i_sa (A)
  Mux : Mux  Inputs=2
  filtroPasaBajos : TransferFcn  Denominator=[1 1]
  is_a : Outport
  Te(Nm) : Outport  Port=2
  wm : Outport  Port=3
  wm1 : Outport  Port=4
  wires:
  filtroPasaBajos/1 -> Mux/1, wm1/1
  Mux/1 -> wm/1
  speed/1 -> Mux/2
  Bus Selector/3 -> is_a/1  "<Stator Current i_sa (A)>"
  Bus Selector/1 -> filtroPasaBajos/1  "<Rotor Speed in (rpm)>"
  m/1 -> Bus Selector/1
  Bus Selector/2 -> 2nd-Order Filter/1  "<Electromagnetic Torque (N*m)>"
  2nd-Order Filter/1 -> Te(Nm)/1

== system MutantsModel2/mutant5/PI Control1 ==
  N* : Inport
  N : Inport  Port=2
  Abs : Abs  SaturateOnIntegerOverflow=on
  Abs1 : Abs  SaturateOnIntegerOverflow=on
  Abs2 : Abs
  Compare To Constant : simulink/Logic and Bit Operations/Compare To Constant  relop=<=  const=0.1  OutDataTypeStr=uint8
  Constant : Constant  Value=0
  Divide : Product  Inputs=/*
  Integrator Limited : Integrator  LimitOutput=on  UpperSaturationLimit=30  LowerSaturationLimit=-30
  Proportional gain : Gain  Gain=0.8  SaturateOnIntegerOverflow=on  OutDataTypeStr=Inherit: Same as input  ParamDataTypeStr=Inherit: Same as input
  Rate Transition3 : RateTransition  OutPortSampleTimeOpt=Inherit
  Saturation : Saturate  UpperLimit=inf  LowerLimit=2
  Saturation2 : Saturate  UpperLimit=120  LowerLimit=0.02
  Sum1 : Sum  Inputs=|+-  SaturateOnIntegerOverflow=on  InputSameDT=on  OutDataTypeStr=Inherit: Same as first input
  Sum2 : Sum  SaturateOnIntegerOverflow=on  InputSameDT=on  OutDataTypeStr=Inherit: Same as first input
  Sum3 : Sum  Inputs=|++  SaturateOnIntegerOverflow=on  InputSameDT=on  OutDataTypeStr=Inherit: Same as first input
  Switch : Switch  Threshold=0.5
  ctrl_sat : Saturate  UpperLimit=30  LowerLimit=-30
  rpm2hz : Gain  Gain=4/120  SaturateOnIntegerOverflow=on  OutDataTypeStr=Inherit: Same as input  ParamDataTypeStr=Inherit: Same as input
  "rpm2hz  " : Gain  Gain=4/120  SaturateOnIntegerOverflow=on  OutDataTypeStr=Inherit: Same as input  ParamDataTypeStr=Inherit: Same as input
  Freq* : Outport
  wires:
  N*/1 -> rpm2hz/1
  Sum2/1 -> ctrl_sat/1
  Sum3/1 -> Saturation2/1
  ctrl_sat/1 -> Sum3/1
  rpm2hz/1 -> Abs/1
  Proportional gain/1 -> Sum2/2
  "rpm2hz  "/1 -> Abs1/1
  Saturation2/1 -> Rate Transition3/1
  Sum1/1 -> Proportional gain/1, Switch/1, Abs2/1
  Abs/1 -> Saturation/1, Sum1/1
  Rate Transition3/1 -> Freq*/1
  Abs1/1 -> Sum3/2, Sum1/2
  N/1 -> "rpm2hz  "/1
  Integrator Limited/1 -> Sum2/1
  Divide/1 -> Compare To Constant/1
  Abs2/1 -> Divide/2
  Compare To Constant/1 -> Switch/2
  Constant/1 -> Switch/3
  Switch/1 -> Integrator Limited/1
  Saturation/1 -> Divide/1

== system MutantsModel2/mutant5/Subsystem ==
  Speed : Inport
  EmergButton1 : Inport  Port=2
  EmergButton2 : Inport  Port=3
  Temperature : Inport  Port=4
  Compare To Constant : simulink/Logic and Bit Operations/Compare To Constant  relop=>  const=100  OutDataTypeStr=boolean
  Compare To Constant1 : simulink/Logic and Bit Operations/Compare To Constant  relop===  const=0  OutDataTypeStr=boolean
  Constant : Constant  Value=emergency_buttons
  Constant1 : Constant  Value=temperature
  Constant2 : Constant  Value=emergency_button2
  Ir_a3 : Scope
  Logical Operator : Logic  Operator=OR  AllPortsSameDT=off  OutDataTypeStr=boolean
  Logical Operator1 : Logic  AllPortsSameDT=off  OutDataTypeStr=boolean
  Logical Operator2 : Logic  AllPortsSameDT=off  OutDataTypeStr=boolean
  Logical Operator3 : Logic  AllPortsSameDT=off  OutDataTypeStr=boolean
  Speed_to_0 : Constant  Value=0
  Switch : Switch  Criteria=u2 ~= 0
  Switch1 : Switch  Criteria=u2 ~= 0
  Switch2 : Switch  Criteria=u2 ~= 0
  Transfer Fcn1 : TransferFcn  Denominator=[20 1]
  "MotorSpeed " : Outport
  wires:
  Transfer Fcn1/1 -> Switch/1
  Compare To Constant1/1 -> Switch2/2
  Switch2/1 -> "MotorSpeed "/1, Ir_a3/1
  Switch1/1 -> Compare To Constant1/1, Switch2/1, Switch2/3
  Constant2/1 -> Logical Operator3/2
  Logical Operator3/1 -> Logical Operator/2
  Logical Operator2/1 -> Switch1/2
  Constant1/1 -> Logical Operator2/2
  Compare To Constant/1 -> Logical Operator2/1
  Temperature/1 -> Compare To Constant/1
  Constant/1 -> Logical Operator1/2
  Logical Operator1/1 -> Switch/2
  Speed_to_0/1 -> Switch/3, Switch1/1
  Switch/1 -> Switch1/3
  Speed/1 -> Transfer Fcn1/1
  Logical Operator/1 -> Logical Operator1/1
  EmergButton2/1 -> Logical Operator3/1
  EmergButton1/1 -> Logical Operator/1

== system MutantsModel2/mutant5/VSI ==
  Freq : Inport
  Fcn : Fcn  Expr=(2*sqrt(2/3)*Vdc/3)*(2*u(1)-u(2)-u(3))
  Fcn1 : Fcn  Expr=(2*sqrt(2/3)*Vdc/3)*(2*u(2)-u(3)-u(1))
  Fcn2 : Fcn  Expr=(2*sqrt(2/3)*Vdc/3)*(2*u(3)-u(2)-u(1))
  SPWM : Subsystem
  Va : Outport
  Vb : Outport  Port=2
  Vc : Outport  Port=3
  wires:
  Freq/1 -> SPWM/1(Freq)
  Fcn/1 -> Va/1
  Fcn2/1 -> Vc/1
  Fcn1/1 -> Vb/1
  SPWM/1(g) -> Fcn1/1, Fcn/1, Fcn2/1

== system MutantsModel2/mutant6/1 HP , 220 V Induction Motor ==
  tau : Inport
  V_a : Inport  Port=2
  V_b : Inport  Port=3
  V_c : Inport  Port=4
  Flux : Subsystem
  Measurements : Subsystem
  Mechanical : Subsystem
  Mux : Mux  Inputs=3
  Mux1 : Mux  Inputs=3
  abc to dq : Subsystem
  d_block : Subsystem
  dq to abc : Subsystem
  "dq to abc " : Subsystem
  q_block : Subsystem
  rad2rpm : Gain  Gain=30/pi
  m : Outport
  wires:
  Mechanical/2(omegaR) -> rad2rpm/1
  Mechanical/3(we) -> Flux/7(we)
  Flux/1(shi_ds) -> d_block/1(shi_ds), Mechanical/1(shi_ds)
  Flux/4("shi_qr ") -> q_block/2(shi_qr)
  d_block/1(i_ds) -> Mechanical/3(i_ds), Measurements/3(I_ds), dq to abc/1(I_d), Flux/3(I_ds)
  d_block/2(i_dr) -> Flux/4(I_dr), "dq to abc "/1(I_d)
  q_block/2(i_qr) -> Measurements/6(I_qr), "dq to abc "/2(I_q), Flux/6(I_qr)
  q_block/1(i_qs) -> Mechanical/4(i_qs), Measurements/4(I_dr), Measurements/5(I_qs), dq to abc/2(I_q), Flux/5(I_qs)
  Mechanical/1(Te) -> Measurements/7(Te)
  tau/1 -> Mechanical/5(tau)
  Flux/2("shi_dr ") -> d_block/2(shi_dr)
  Flux/3(shi_qs) -> q_block/1(shi_qs), Mechanical/2(shi_qs)
  abc to dq/1(V_ds) -> Flux/1(V_ds)
  abc to dq/2(V_qs) -> Flux/2(V_qs)
  V_c/1 -> abc to dq/3(Vc)
  V_b/1 -> abc to dq/2(Vb)
  V_a/1 -> abc to dq/1(Va)
  dq to abc/1(i_sa) -> Mux/1
  "dq to abc "/1(i_ra) -> Mux1/1
  dq to abc/2(i_sb) -> Mux/2
  dq to abc/3(i_sc) -> Mux/3
  "dq to abc "/3(i_rc) -> Mux1/3
  "dq to abc "/2(i_rb) -> Mux1/2
  Mux/1 -> Measurements/1(I_s)
  Mux1/1 -> Measurements/2(I_r)
  rad2rpm/1 -> Measurements/8(N)
  Measurements/1(m) -> m/1

== system MutantsModel2/mutant6/Data Acquision ==
  note: DONE TO HAVE AN ALLOWABLE SIMULATION TIME
  m : Inport
  speed : Inport  Port=2
  2nd-Order Filter : powerlib_extras/Control  Blocks/2nd-Order Filter  FilterType=Lowpass  Fo=120  Zeta=0.707  Initialize=off  Vac_Init=[1 45 60]  Vdc_Init=-0.5  PlotResponse=off  param1=[1 500 1]
  Bus Selector : BusSelector  OutputSignals=Mechanical.Rotor Speed in (rpm),Mechanical.Electromagnetic Torque (N*m),Stator Measurement.Stator Current i_sa (A)
  Mux : Mux  Inputs=2
  filtroPasaBajos : TransferFcn  Denominator=[1 1]
  is_a : Outport
  Te(Nm) : Outport  Port=2
  wm : Outport  Port=3
  wm1 : Outport  Port=4
  wires:
  2nd-Order Filter/1 -> Te(Nm)/1
  Bus Selector/2 -> 2nd-Order Filter/1  "<Electromagnetic Torque (N*m)>"
  m/1 -> Bus Selector/1
  Bus Selector/1 -> filtroPasaBajos/1  "<Rotor Speed in (rpm)>"
  Bus Selector/3 -> is_a/1  "<Stator Current i_sa (A)>"
  speed/1 -> Mux/2
  Mux/1 -> wm/1
  filtroPasaBajos/1 -> wm1/1, Mux/1

== system MutantsModel2/mutant6/PI Control1 ==
  N* : Inport
  N : Inport  Port=2
  Abs : Abs  SaturateOnIntegerOverflow=on
  Abs1 : Abs  SaturateOnIntegerOverflow=on
  Abs2 : Abs
  Compare To Constant : simulink/Logic and Bit Operations/Compare To Constant  relop=<=  const=0.1  OutDataTypeStr=uint8
  Constant : Constant  Value=0
  Divide : Product  Inputs=/*
  Integrator Limited : Integrator  LimitOutput=on  UpperSaturationLimit=30  LowerSaturationLimit=-30
  Proportional gain : Gain  Gain=0.8  SaturateOnIntegerOverflow=on  OutDataTypeStr=Inherit: Same as input  ParamDataTypeStr=Inherit: Same as input
  Rate Transition3 : RateTransition  OutPortSampleTimeOpt=Inherit
  Saturation : Saturate  UpperLimit=inf  LowerLimit=2
  Saturation2 : Saturate  UpperLimit=120  LowerLimit=0.02
  Sum1 : Sum  Inputs=|+-  SaturateOnIntegerOverflow=on  InputSameDT=on  OutDataTypeStr=Inherit: Same as first input
  Sum2 : Sum  SaturateOnIntegerOverflow=on  InputSameDT=on  OutDataTypeStr=Inherit: Same as first input
  Sum3 : Sum  Inputs=|++  SaturateOnIntegerOverflow=on  InputSameDT=on  OutDataTypeStr=Inherit: Same as first input
  Switch : Switch  Threshold=0.5
  ctrl_sat : Saturate  UpperLimit=30  LowerLimit=-30
  rpm2hz : Gain  Gain=4/120  SaturateOnIntegerOverflow=on  OutDataTypeStr=Inherit: Same as input  ParamDataTypeStr=Inherit: Same as input
  "rpm2hz  " : Gain  Gain=4/120  SaturateOnIntegerOverflow=on  OutDataTypeStr=Inherit: Same as input  ParamDataTypeStr=Inherit: Same as input
  Freq* : Outport
  wires:
  Saturation/1 -> Divide/1
  Switch/1 -> Integrator Limited/1
  Constant/1 -> Switch/3
  Compare To Constant/1 -> Switch/2
  Abs2/1 -> Divide/2
  Divide/1 -> Compare To Constant/1
  Integrator Limited/1 -> Sum2/1
  N/1 -> "rpm2hz  "/1
  Abs1/1 -> Sum1/2, Sum3/2
  Rate Transition3/1 -> Freq*/1
  Abs/1 -> Sum1/1, Saturation/1
  Sum1/1 -> Abs2/1, Switch/1, Proportional gain/1
  Saturation2/1 -> Rate Transition3/1
  "rpm2hz  "/1 -> Abs1/1
  Proportional gain/1 -> Sum2/2
  rpm2hz/1 -> Abs/1
  ctrl_sat/1 -> Sum3/1
  Sum3/1 -> Saturation2/1
  Sum2/1 -> ctrl_sat/1
  N*/1 -> rpm2hz/1

== system MutantsModel2/mutant6/Subsystem ==
  Speed : Inport
  EmergButton1 : Inport  Port=2
  EmergButton2 : Inport  Port=3
  Temperature : Inport  Port=4
  Compare To Constant : simulink/Logic and Bit Operations/Compare To Constant  relop=>  const=100  OutDataTypeStr=boolean
  Compare To Constant1 : simulink/Logic and Bit Operations/Compare To Constant  relop=>=  const=0  OutDataTypeStr=boolean
  Constant : Constant  Value=emergency_buttons
  Constant1 : Constant  Value=temperature
  Constant2 : Constant  Value=emergency_button2
  Ir_a3 : Scope
  Logical Operator : Logic  Operator=OR  AllPortsSameDT=off  OutDataTypeStr=boolean
  Logical Operator1 : Logic  AllPortsSameDT=off  OutDataTypeStr=boolean
  Logical Operator2 : Logic  AllPortsSameDT=off  OutDataTypeStr=boolean
  Logical Operator3 : Logic  AllPortsSameDT=off  OutDataTypeStr=boolean
  Speed_to_0 : Constant  Value=0
  Switch : Switch  Criteria=u2 ~= 0
  Switch1 : Switch  Criteria=u2 ~= 0
  Switch2 : Switch  Criteria=u2 ~= 0
  Transfer Fcn1 : TransferFcn  Denominator=[20 1]
  "MotorSpeed " : Outport
  wires:
  EmergButton1/1 -> Logical Operator/1
  EmergButton2/1 -> Logical Operator3/1
  Logical Operator/1 -> Logical Operator1/1
  Speed/1 -> Transfer Fcn1/1
  Switch/1 -> Switch1/3
  Speed_to_0/1 -> Switch1/1, Switch/1
  Logical Operator1/1 -> Switch/2
  Constant/1 -> Logical Operator1/2
  Temperature/1 -> Compare To Constant/1
  Compare To Constant/1 -> Logical Operator2/1
  Constant1/1 -> Logical Operator2/2
  Logical Operator2/1 -> Switch1/2
  Logical Operator3/1 -> Logical Operator/2
  Constant2/1 -> Logical Operator3/2
  Switch1/1 -> Switch2/3, Switch2/1, Compare To Constant1/1
  Switch2/1 -> Ir_a3/1, "MotorSpeed "/1
  Compare To Constant1/1 -> Switch2/2
  Transfer Fcn1/1 -> Switch/3

== system MutantsModel2/mutant6/VSI ==
  Freq : Inport
  Fcn : Fcn  Expr=(2*sqrt(2/3)*Vdc/3)*(2*u(1)-u(2)-u(3))
  Fcn1 : Fcn  Expr=(2*sqrt(2/3)*Vdc/3)*(2*u(2)-u(3)-u(1))
  Fcn2 : Fcn  Expr=(2*sqrt(2/3)*Vdc/3)*(2*u(3)-u(2)-u(1))
  SPWM : Subsystem
  Va : Outport
  Vb : Outport  Port=2
  Vc : Outport  Port=3
  wires:
  SPWM/1(g) -> Fcn2/1, Fcn/1, Fcn1/1
  Fcn1/1 -> Vb/1
  Fcn2/1 -> Vc/1
  Fcn/1 -> Va/1
  Freq/1 -> SPWM/1(Freq)

== system MutantsModel2/mutant7/1 HP , 220 V Induction Motor ==
  tau : Inport
  V_a : Inport  Port=2
  V_b : Inport  Port=3
  V_c : Inport  Port=4
  Flux : Subsystem
  Measurements : Subsystem
  Mechanical : Subsystem
  Mux : Mux  Inputs=3
  Mux1 : Mux  Inputs=3
  abc to dq : Subsystem
  d_block : Subsystem
  dq to abc : Subsystem
  "dq to abc " : Subsystem
  q_block : Subsystem
  rad2rpm : Gain  Gain=30/pi
  m : Outport
  wires:
  Mechanical/2(omegaR) -> rad2rpm/1
  Mechanical/3(we) -> Flux/7(we)
  Flux/1(shi_ds) -> d_block/1(shi_ds), Mechanical/1(shi_ds)
  Flux/4("shi_qr ") -> q_block/2(shi_qr)
  d_block/1(i_ds) -> Mechanical/3(i_ds), Measurements/3(I_ds), dq to abc/1(I_d), Flux/3(I_ds)
  d_block/2(i_dr) -> Flux/4(I_dr), "dq to abc "/1(I_d)
  q_block/2(i_qr) -> Measurements/6(I_qr), "dq to abc "/2(I_q), Flux/6(I_qr)
  q_block/1(i_qs) -> Mechanical/4(i_qs), Measurements/4(I_dr), Measurements/5(I_qs), dq to abc/2(I_q), Flux/5(I_qs)
  Mechanical/1(Te) -> Measurements/7(Te)
  tau/1 -> Mechanical/5(tau)
  Flux/2("shi_dr ") -> d_block/2(shi_dr)
  Flux/3(shi_qs) -> q_block/1(shi_qs), Mechanical/2(shi_qs)
  abc to dq/1(V_ds) -> Flux/1(V_ds)
  abc to dq/2(V_qs) -> Flux/2(V_qs)
  V_c/1 -> abc to dq/3(Vc)
  V_b/1 -> abc to dq/2(Vb)
  V_a/1 -> abc to dq/1(Va)
  dq to abc/1(i_sa) -> Mux/1
  "dq to abc "/1(i_ra) -> Mux1/1
  dq to abc/2(i_sb) -> Mux/2
  dq to abc/3(i_sc) -> Mux/3
  "dq to abc "/3(i_rc) -> Mux1/3
  "dq to abc "/2(i_rb) -> Mux1/2
  Mux/1 -> Measurements/1(I_s)
  Mux1/1 -> Measurements/2(I_r)
  rad2rpm/1 -> Measurements/8(N)
  Measurements/1(m) -> m/1

== system MutantsModel2/mutant7/Data Acquision ==
  note: DONE TO HAVE AN ALLOWABLE SIMULATION TIME
  m : Inport
  speed : Inport  Port=2
  2nd-Order Filter : powerlib_extras/Control  Blocks/2nd-Order Filter  FilterType=Lowpass  Fo=120  Zeta=0.707  Initialize=off  Vac_Init=[1 45 60]  Vdc_Init=-0.5  PlotResponse=off  param1=[1 500 1]
  Bus Selector : BusSelector  OutputSignals=Mechanical.Rotor Speed in (rpm),Mechanical.Electromagnetic Torque (N*m),Stator Measurement.Stator Current i_sa (A)
  Mux : Mux  Inputs=2
  filtroPasaBajos : TransferFcn  Denominator=[1 1]
  is_a : Outport
  Te(Nm) : Outport  Port=2
  wm : Outport  Port=3
  wm1 : Outport  Port=4
  wires:
  2nd-Order Filter/1 -> Te(Nm)/1
  Bus Selector/2 -> 2nd-Order Filter/1  "<Electromagnetic Torque (N*m)>"
  m/1 -> Bus Selector/1
  Bus Selector/1 -> filtroPasaBajos/1  "<Rotor Speed in (rpm)>"
  Bus Selector/3 -> is_a/1  "<Stator Current i_sa (A)>"
  speed/1 -> Mux/2
  Mux/1 -> wm/1
  filtroPasaBajos/1 -> wm1/1, Mux/1
